simulink model "UnmodifiedMotoHawkModel"  (R2016a)
settings: Solver=ode4  SolverMode=SingleTasking  StartTime=0.0  StopTime=10.0  FixedStep=0.001  RelTol=1e-3
values from neighbouring files (symbols this model uses):
  engineblendfactormap = [0 0 0 0 0 0 0 0 0 0 0 0 ... (420 elements, 21x20)]    [blendfactorvariables.mat]
  motorblendfactormap = [1 1 1 1 1 1 1 1 1 1 1 1 ... (420 elements, 21x20)]    [blendfactorvariables.mat]
  v = [0 5 10 15 20 25 30 35 40 45 50 55 ... (21 elements, 1x21)]    [blendfactorvariables.mat]
  x = [0 1 2 3 4 5 6 7 8 9 10 11 ... (20 elements, 1x20)]    [blendfactorvariables.mat]
undefined symbols (not defined in the file or in its folder): ECU565, motohawk_build_version, motohawk_trunc_name, motohawk_vardec_path
libraries: MotoHawk_lib x58
(part 1 of 2)
settings Model: MotoHawkModelGUID=5F89A2C4-B071-4908-A4AC-2A815C8EF35E  MotoHawkModelOpenTime=2017 4 23 0 12 7.93  MotoHawkBuildVersion=014  MotoHawkBuildStats=struct('TotalFLASH',{0},'TotalEEPROM',{0},'TotalRAM',{0},'AppFLASH',{0},'AppEEPROM',{0},'AppRAM',{0},'HeapRAM',{0},'BuildSuccessCount',{14},'BuildErrorCount',{14})  MotoHawkBuildDirectory=C:\Users\Saumya Trivedi\Documents\MTU\2nd Semester\5750 - Distributed Embedded Control System\Lab\Final Project\Final Models After Testing-20170418T230125Z-001\Final Models After Testing\UnmodifiedMotoHawkModel_Build  MotoHawkBuildInfo=struct('refmodel',{0},'model_name',{'UnmodifiedMotoHawkModel'},'motohawk_version',{'2016a_sp1.1722'},'motohawk_component_version',{'0.0.8'},'motohawk_refmdl_version',{'0.0.1'},'matlab_version',{'9.0.0'},'build_version',{'013'},'module_type',{'ECU565-128'},'layout_type',{'DEV'},'enable_build',{1},'processor_family',{'PPC'},'processor_type',{'MPC565'},'toolchain_vendor',{'gcc-powerpc-eabi'},'toolchain_version',{'4.6.0'},'component',{0},'archive_file',{'PCM128.a'},'fptype',{0},'flash_size',{1048576},'ee_size',{8192},'ram_size',{36864},'decram_size',{4096},'eri_table0_rev',{12},'max_eri_table_size',{65535},'fgnd_base_period_ms',{5},'bgnd_base_period_ms',{50},'build_dir',{'H:\Desktop\5750 Final Project\Final Models\Final Models\UnmodifiedMotoHawkModel_Build'},'dll_name',{'UnmodifiedMotoHawkModel_013'},'srz_name',{'UnmodifiedMotoHawkModel_013'},'fgnd_stack_size',{3072},'fgnd_angle_stack_size',{0},'bgnd_stack_size',{2048},'idle_stack_size',{1024},'irq_stack_size',{1536},'irq_stack_margin',{153},'heap_size',{4096},'heap_margin',{409},'app_int_stack_size',{1024},'shutdown_stack_size',{1024},'use_target_os_config',{0},'target_os',{'Classic ControlCore'},'install_dll_dir',{'C:\ECUFiles\TDBDLL'},'install_srz_dir',{'C:\ECUFiles\Programs'},'mingw_dir',{'C:\Program Files (x86)\Woodward\DevelopmentTools\Toolchains\GCC\win32-pe\4_7_0'},'motohawk_dir',{'C:\Program Files (x86)\Woodward\MCS\MotoHawk\2016a_sp1.1722'},'toolchain_dir',{'C:\Program Files (x86)\Woodward\DevelopmentTools\Toolchains\GCC\powerpc-eabi\4_6_0'},'matlab_root',{'C:\Program Files\MATLAB\R2016a'},'model_guid',{'5F89A2C4-B071-4908-A4AC-2A815C8EF35E'},'build_guid',{'792EB62F-FFF4-451D-B1A3-A5F3AFC705B8'},'token_guid',{'276056F1851C404EAF8E31A6D21D1C4E'})  MotoHawkModelSavedName=UnmodifiedMotoHawkModel  MotoHawkModelElapsedTime=579139.132  MotoHawkBuildGUID=792EB62F-FFF4-451D-B1A3-A5F3AFC705B8  Creator=vaibhav  LastModifiedBy=Saumya Trivedi
settings ConfigSet: Description="This Simulink Configuration Set is preconfigured  for the MotoHawk target \"ECU565-128\"."
settings OptimizationCC: DefaultParameterBehavior=Inlined  InlineInvariantSignals=on  EnhancedBackFolding=on  InitFltsAndDblsToZero=on  NoFixptDivByZeroProtection=on  EfficientFloat2IntCast=on  OptimizeModelRefInitCode=on  LifeSpan=1
settings DebuggingCC: InheritedTsInSrcMsg=none  TasksWithSamePriorityMsg=none  ParameterTunabilityLossMsg=error  ModelReferenceIOMismatchMessage=warning  SFUnexpectedBacktrackingDiag=error  SFNoUnconditionalDefaultTransitionDiag=error
settings HardwareCC: ProdBitPerPointer=32  ProdLargestAtomicInteger=Integer  ProdIntDivRoundTo=Undefined  ProdEndianess=BigEndian  ProdWordSize=32  ProdHWDeviceType=Specified
settings ModelReferenceCC: UpdateModelReferenceTargets=IfOutOfDate  CheckModelReferenceTargetMessage=warning  ModelReferenceNumInstancesAllowed=Single
settings RTWCC: SystemTargetFile=motohawk_ert_rtw.tlc  MakeCommand=make_rtw_motohawk  TemplateMakefile=motohawk_ert_rtw.tmf  Description=MotoHawk(tm) Rapid Prototyping  GenerateReport=on  IncludeHyperlinkInReport=on  LaunchReport=on  GenerateTraceInfo=on  GenerateTraceReport=on  GenerateTraceReportSl=on  GenerateTraceReportSf=on  GenerateTraceReportEml=on
settings CodeAppCC: ForceParamTrailComments=on  IgnoreCustomStorageClasses=off  MaxIdLength=100  OperatorAnnotations=on  SimulinkDataObjDesc=on  SFDataObjDesc=on  MATLABFcnDesc=on  CustomSymbolStrType=$N$R$M  CustomSymbolStrField=$H$N$M  InsertBlockDesc=on  MATLABSourceComments=on  InternalIdentifier=Classic
settings STFCustomTargetCC: TargetLangStandard=C99 (ISO)  ERTMultiwordTypeDef=User defined  ERTMultiwordLength=0  IncludeMdlTerminateFcn=off  GeneratePreprocessorConditionals=Disable all  CombineOutputUpdateFcns=on  SuppressErrorStatus=on  ERTCustomFileBanners=on  SupportContinuousTime=off  SupportNonInlinedSFcns=off  MATLABClassNameForMDSCustomization=Simulink.SoftwareTarget.ERTCustomization  GRTInterface=off  SystemTargetFile=motohawk_ert_rtw.tlc
settings ERTTargetCC: TargetLangStandard=C99 (ISO)  ERTMultiwordTypeDef=User defined  ERTMultiwordLength=0  ParMdlRefBuildCompliant=off  CompOptLevelCompliant=off  ConcurrentExecutionCompliant=off  IncludeMdlTerminateFcn=off  GeneratePreprocessorConditionals=Disable all  SuppressErrorStatus=on  ERTFirstTimeCompliant=off  ModelStepFunctionPrototypeControlCompliant=off  CPPClassGenCompliant=off  UseToolchainInfoCompliant=off  InlinedParameterPlacement=NonHierarchical  ERTCustomFileTemplate=motohawk_file_process.tlc
settings ConfigComp: CovMetricSettings=dwe  CovHtmlReporting=off  CovSaveCumulativeToWorkspaceVar=off  CovSaveSingleToWorkspaceVar=off  CovExternalEMLEnable=on

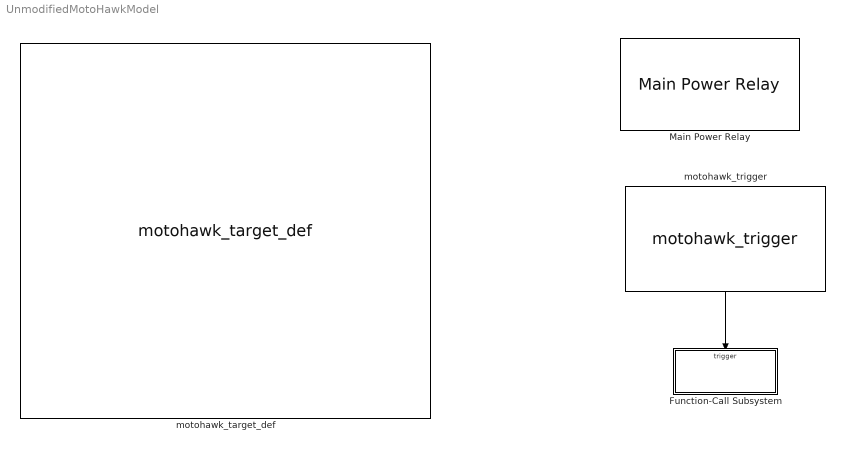
== system UnmodifiedMotoHawkModel ==
  Function-Call Subsystem : Subsystem  TreatAsAtomicUnit=on
  Main Power Relay : MotoHawk_lib/Extra Development Blocks/Main Power Relay  on_delay_count=2  off_delay_count=5  ecup_threshold=100  group='System | Main Power Relay'
  motohawk_target_def : MotoHawk_lib/motohawk_target_def  Priority=-65535  target=ECU565-128  layout=DEV  fptype=single (32 bits)  use_target_os_config=off  target_os=ControlCore  default_target_os=Classic ControlCore  fgnd_stack_size=3*1024  fgnd_angle_stack_size=0  bgnd_stack_size=2*1024  idle_stack_size=1024  irq_stack_size=1536  app_int_stack_size=1024  shutdown_stack_size=1024  heap_size=4*1024  show_margins=off  fgnd_stack_margin=(3*1024) * 0.1  fgnd_angle_stack_margin=0  bgnd_stack_margin=(2*1024) * 0.1  idle_stack_margin=(1024) * 0.1  irq_stack_margin=(1536) * 0.1  app_int_stack_margin=(1024) * 0.1  shutdown_stack_margin=(1024) * 0.1  heap_margin=(4*1024) * 0.1  comp_name=bdroot  comp_img='KVASER_CAN_USB.jpg'  comp_security=No Encryption  comp_build_pass='mhbuild'  comp_sim_pass='mhsim'  comp_multi=off  show_filenames=off  dll_name=motohawk_trunc_name(bdroot, ['_' motohawk_build_version], 50)  srz_name=motohawk_trunc_name(bdroot, ['_' motohawk_build_version], 50)  build_dir='.'  comp_dir='.'
  motohawk_trigger : MotoHawk_lib/Trigger Blocks/motohawk_trigger  Tag=Trigger  Priority=0  trig_name=[]  trigger=FGND_RTI_PERIODIC  priority_order=0  inherited=off  run_disabled=off  override_app_monitor=off  target=ECU565_128
  wires:
  motohawk_trigger/1 -> Function-Call Subsystem/Trigger

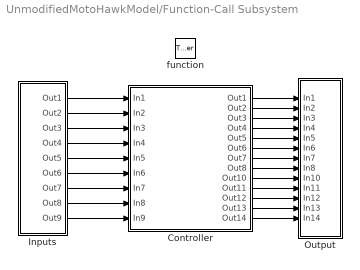
== system UnmodifiedMotoHawkModel/Function-Call Subsystem ==
  function : TriggerPort  TriggerType=function-call  VariantControl=Variant
  Controller : Subsystem
  Inputs : Subsystem
  Output : Subsystem
  wires:
  Inputs/1(Out1) -> Controller/1(In1)
  Inputs/2(Out2) -> Controller/2(In2)
  Inputs/3(Out3) -> Controller/3(In3)
  Inputs/4(Out4) -> Controller/4(In4)
  Inputs/5(Out5) -> Controller/5(In5)
  Inputs/6(Out6) -> Controller/6(In6)
  Inputs/7(Out7) -> Controller/7(In7)
  Inputs/8(Out8) -> Controller/8(In8)
  Inputs/9(Out9) -> Controller/9(In9)
  Controller/1(Out1) -> Output/1(In1)
  Controller/2(Out2) -> Output/2(In2)
  Controller/3(Out3) -> Output/3(In3)
  Controller/4(Out4) -> Output/4(In4)
  Controller/5(Out5) -> Output/5(In5)
  Controller/6(Out6) -> Output/6(In6)
  Controller/7(Out7) -> Output/7(In7)
  Controller/8(Out8) -> Output/8(In8)
  Controller/9(Out10) -> Output/9(In10)
  Controller/10(Out11) -> Output/10(In11)
  Controller/11(Out12) -> Output/11(In12)
  Controller/12(Out13) -> Output/12(In13)
  Controller/13(Out14) -> Output/13(In14)

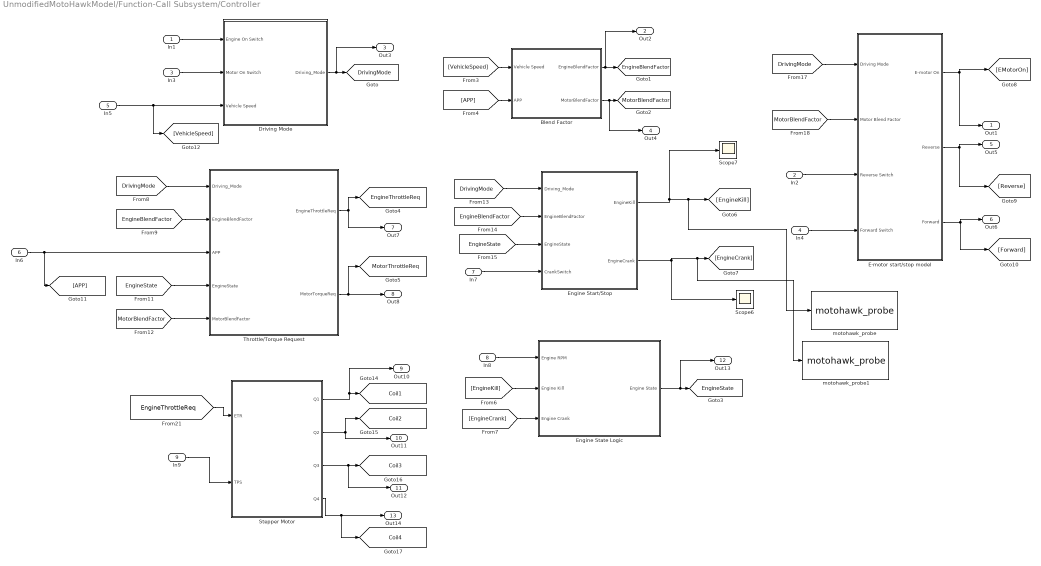
== system UnmodifiedMotoHawkModel/Function-Call Subsystem/Controller ==
  In1 : Inport
  In2 : Inport  Port=2
  In3 : Inport  Port=3
  In4 : Inport  Port=4
  In5 : Inport  Port=5
  In6 : Inport  Port=6
  In7 : Inport  Port=7
  In8 : Inport  Port=8
  In9 : Inport  Port=9
  Blend Factor : Subsystem
  Driving Mode : Subsystem
  E-motor start/stop model : Subsystem
  Engine Start/Stop : Subsystem
  Engine State Logic : Subsystem
  Scope6 : Scope
  Scope7 : Scope
  Stepper Motor : Subsystem
  Throttle/Torque Request : Subsystem
  motohawk_probe : MotoHawk_lib/Calibration & Probing Blocks/motohawk_probe  nam='EngineKill'  show_more=off  name_source=Use Parameter  read_level=1  view_as=Number  enum_struct={'Disabled', 'Enabled'}  vector_style=Wide Row  use_help_units=off  help=''  units=''  use_header_enum=off  row_header_enum={}  col_header_enum={}  use_min_max=off  min_val=-inf  max_val=inf  use_precision=off  precision=''  gain=1  offset=0  exp=1  use_mototune_group=off  mototune_group=motohawk_vardec_path(gcb)
  motohawk_probe1 : MotoHawk_lib/Calibration & Probing Blocks/motohawk_probe  nam='EngineCrank'  show_more=off  name_source=Use Parameter  read_level=1  view_as=Number  enum_struct={'Disabled', 'Enabled'}  vector_style=Wide Row  use_help_units=off  help=''  units=''  use_header_enum=off  row_header_enum={}  col_header_enum={}  use_min_max=off  min_val=-inf  max_val=inf  use_precision=off  precision=''  gain=1  offset=0  exp=1  use_mototune_group=off  mototune_group=motohawk_vardec_path(gcb)
  Out1 : Outport
  Out2 : Outport  Port=2
  Out3 : Outport  Port=3
  Out4 : Outport  Port=4
  Out5 : Outport  Port=5
  Out6 : Outport  Port=6
  Out7 : Outport  Port=7
  Out8 : Outport  Port=8
  Out10 : Outport  Port=9
  Out11 : Outport  Port=10
  Out12 : Outport  Port=11
  Out13 : Outport  Port=12
  Out14 : Outport  Port=13
  tag scope: Coil1=global, Coil2=global, Coil3=global, Coil4=global, DrivingMode=global, EngineBlendFactor=global, EngineState=global, EngineThrottleReq=global, MotorBlendFactor=global, MotorThrottleReq=global
  wires:
  Driving Mode/1(Driving_Mode) -> Out3/1, [DrivingMode]
  [VehicleSpeed] -> Blend Factor/1(Vehicle Speed)
  [APP] -> Blend Factor/2(APP)
  Blend Factor/2(MotorBlendFactor) -> Out4/1, [MotorBlendFactor]
  [EngineCrank] -> Engine State Logic/3(Engine Crank)
  [EngineKill] -> Engine State Logic/2(Engine Kill)
  Engine State Logic/1(Engine State) -> Out13/1, [EngineState]
  [DrivingMode] -> Throttle/Torque Request/1(Driving_Mode)
  [EngineBlendFactor] -> Throttle/Torque Request/2(EngineBlendFactor)
  Blend Factor/1(EngineBlendFactor) -> Out2/1, [EngineBlendFactor]
  E-motor start/stop model/2(Reverse) -> Out5/1, [Reverse]
  E-motor start/stop model/1(E-motor On) -> [EMotorOn], Out1/1
  [EngineState] -> Throttle/Torque Request/4(EngineState)
  [MotorBlendFactor] -> Throttle/Torque Request/5(MotorBlendFactor)
  Throttle/Torque Request/1(EngineThrottleReq) -> Out7/1, [EngineThrottleReq]
  Throttle/Torque Request/2(MotorTorqueReq) -> [MotorThrottleReq], Out8/1
  [DrivingMode] -> Engine Start/Stop/1(Driving_Mode)
  [EngineBlendFactor] -> Engine Start/Stop/2(EngineBlendFactor)
  [EngineState] -> Engine Start/Stop/3(EngineState)
  Engine Start/Stop/1(EngineKill) -> Scope7/1, motohawk_probe/1, [EngineKill]
  [DrivingMode] -> E-motor start/stop model/1(Driving Mode)
  E-motor start/stop model/3(Forward) -> Out6/1, [Forward]
  [EngineThrottleReq] -> Stepper Motor/1(ETR)
  Stepper Motor/1(Q1) -> Out10/1, [Coil1]
  Stepper Motor/4(Q4) -> [Coil4], Out14/1
  Stepper Motor/3(Q3) -> Out12/1, [Coil3]
  Stepper Motor/2(Q2) -> [Coil2], Out11/1
  [MotorBlendFactor] -> E-motor start/stop model/2(Motor Blend Factor)
  Engine Start/Stop/2(EngineCrank) -> motohawk_probe1/1, [EngineCrank], Scope6/1
  In4/1 -> E-motor start/stop model/4(Forward Switch)
  In2/1 -> E-motor start/stop model/3(Reverse Switch)
  In3/1 -> Driving Mode/2(Motor On Switch)
  In1/1 -> Driving Mode/1(Engine On Switch)
  In9/1 -> Stepper Motor/2(TPS)
  In8/1 -> Engine State Logic/1(Engine RPM)
  In7/1 -> Engine Start/Stop/4(CrankSwitch)
  In5/1 -> [VehicleSpeed], Driving Mode/3(Vehicle Speed)
  In6/1 -> Throttle/Torque Request/3(APP), [APP]

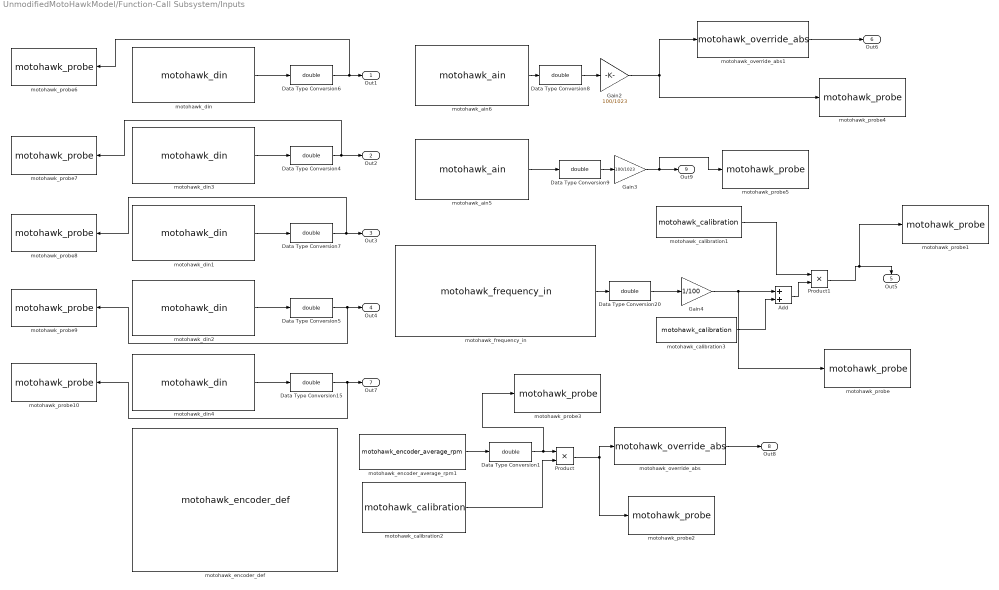
== system UnmodifiedMotoHawkModel/Function-Call Subsystem/Inputs ==
  Add : Sum
  Data Type Conversion{1,4..9,15,20} (9 alike) : DataTypeConversion  OutDataTypeStr=double
  Gain2 : Gain  Gain=100/1023
  Gain3 : Gain  Gain=100/1023
  Gain4 : Gain  Gain=1/100
  Product : Product
  Product1 : Product
  motohawk_ain5 : MotoHawk_lib/Analog I//O Blocks/motohawk_ain  res_name=['TPS']  text_resource=AN25M  code_resource=NONE  val_resource=-1  target=ECU565-128  resource_enum_str=(None)=-1,ECUP=53,DRVP=54,XDRP=55,AN1M=56,AN2M=57,AN3M=58,AN4M=59,AN5M=60,AN6M=61,AN7M=62,AN8M=63,AN9M=64,AN10M=65,AN11M=66,AN12M=67,AN13M=68,AN14M=69,AN15M=70,AN16M=71,AN17M=72,AN18M=73,AN19M=74,AN20M=75,AN21M=76,AN22M=77,AN23M=78,AN24M=79,AN25M=80,AN26M=81,AN27M=82,AN28M=83,AN29M=84,AN30M=85,AN31M=86,AN32M=87,AN33M=88,AN34M=89,O2A=90,O2B=91,XDRP_B=92,REF_14V=143  altref=5V Reference  typ=uint16  num_adc_bits=10  use_stat=off  use_vardec=off  nam='RTD1_MW'  read_level=1  write_level=1  group='System | I/O Pins | Inputs Config'
  motohawk_ain6 : MotoHawk_lib/Analog I//O Blocks/motohawk_ain  res_name=['APP']  text_resource=AN22M  code_resource=NONE  val_resource=-1  target=ECU565-128  resource_enum_str=(None)=-1,ECUP=53,DRVP=54,XDRP=55,AN1M=56,AN2M=57,AN3M=58,AN4M=59,AN5M=60,AN6M=61,AN7M=62,AN8M=63,AN9M=64,AN10M=65,AN11M=66,AN12M=67,AN13M=68,AN14M=69,AN15M=70,AN16M=71,AN17M=72,AN18M=73,AN19M=74,AN20M=75,AN21M=76,AN22M=77,AN23M=78,AN24M=79,AN25M=80,AN26M=81,AN27M=82,AN28M=83,AN29M=84,AN30M=85,AN31M=86,AN32M=87,AN33M=88,AN34M=89,O2A=90,O2B=91,XDRP_B=92,REF_14V=143  altref=5V Reference  typ=uint16  num_adc_bits=10  use_stat=off  use_vardec=off  nam='RTD1_MW'  read_level=1  write_level=1  group='System | I/O Pins | Inputs Config'
  motohawk_calibration1 : MotoHawk_lib/Calibration & Probing Blocks/motohawk_calibration  nam='Speed_Gain'  val=1  storage=Calibration  show_more=off  name_source=Use Parameter  data_type=Inherit from 'Default Value'  read_level=1  write_level=1  ovr_cals=on  view_as=Number  enum_struct={'Disabled', 'Enabled'}  vector_style=Wide Row  use_help_units=off  help=''  units=''  use_header_enum=off  row_header_enum={}  col_header_enum={}  use_min_max=off  min_val=-inf  max_val=inf  use_precision=off  precision=''  gain=1  offset=0  exp=1  use_mototune_group=off  mototune_group=motohawk_vardec_path(gcb)  data_stores=motohawk_sfun_calibration_data_stores
  motohawk_calibration2 : MotoHawk_lib/Calibration & Probing Blocks/motohawk_calibration  nam='Rpm_Gain'  val=1  storage=Calibration  show_more=off  name_source=Use Parameter  data_type=Inherit from 'Default Value'  read_level=1  write_level=1  ovr_cals=on  view_as=Number  enum_struct={'Disabled', 'Enabled'}  vector_style=Wide Row  use_help_units=off  help=''  units=''  use_header_enum=off  row_header_enum={}  col_header_enum={}  use_min_max=off  min_val=-inf  max_val=inf  use_precision=off  precision=''  gain=1  offset=0  exp=1  use_mototune_group=off  mototune_group=motohawk_vardec_path(gcb)  data_stores=motohawk_sfun_calibration_data_stores
  motohawk_calibration3 : MotoHawk_lib/Calibration & Probing Blocks/motohawk_calibration  nam='Speed_Offset'  val=1  storage=Calibration  show_more=off  name_source=Use Parameter  data_type=Inherit from 'Default Value'  read_level=1  write_level=1  ovr_cals=on  view_as=Number  enum_struct={'Disabled', 'Enabled'}  vector_style=Wide Row  use_help_units=off  help=''  units=''  use_header_enum=off  row_header_enum={}  col_header_enum={}  use_min_max=off  min_val=-inf  max_val=inf  use_precision=off  precision=''  gain=1  offset=0  exp=1  use_mototune_group=off  mototune_group=motohawk_vardec_path(gcb)  data_stores=motohawk_sfun_calibration_data_stores
  motohawk_din : MotoHawk_lib/Digital I//O Blocks/motohawk_din  resource_name=['EngineOnSwitch']  text_resource=AN5M  code_resource=NONE  val_resource=-1  target=ECU565-128  resource_enum_str=(None)=-1,AN1M=56,AN2M=57,AN3M=58,AN4M=59,AN5M=60,AN6M=61,AN7M=62,AN8M=63,AN9M=64,AN10M=65,AN11M=66,AN12M=67,AN13M=68,AN14M=69,AN15M=70,AN16M=71,AN17M=72,AN18M=73,AN19M=74,AN20M=75,AN21M=76,AN22M=77,AN23M=78,AN24M=79,AN25M=80,AN26M=81,AN27M=82,AN28M=83,AN29M=84,AN30M=85,AN31M=86,AN32M=87,AN33M=88,AN34M=89,O2A=90,O2B=91,DG1M=93,DG2M=94,DG3M=95,DG4M=96,DG5M=102,DG6M=103,DG7M=104,SPD1=105,SPD2=106,DG8M=111  pullup=None  use_stat=off  use_vardec=off  nam=[]  read_level=1  write_level=1  group='System | I/O Pins | Inputs Config'
  motohawk_din1 : MotoHawk_lib/Digital I//O Blocks/motohawk_din  resource_name=['MotorOnSwitch']  text_resource=AN6M  code_resource=NONE  val_resource=-1  target=ECU565-128  resource_enum_str=(None)=-1,AN1M=56,AN2M=57,AN3M=58,AN4M=59,AN5M=60,AN6M=61,AN7M=62,AN8M=63,AN9M=64,AN10M=65,AN11M=66,AN12M=67,AN13M=68,AN14M=69,AN15M=70,AN16M=71,AN17M=72,AN18M=73,AN19M=74,AN20M=75,AN21M=76,AN22M=77,AN23M=78,AN24M=79,AN25M=80,AN26M=81,AN27M=82,AN28M=83,AN29M=84,AN30M=85,AN31M=86,AN32M=87,AN33M=88,AN34M=89,O2A=90,O2B=91,DG1M=93,DG2M=94,DG3M=95,DG4M=96,DG5M=102,DG6M=103,DG7M=104,SPD1=105,SPD2=106,DG8M=111  pullup=None  use_stat=off  use_vardec=off  nam=[]  read_level=1  write_level=1  group='System | I/O Pins | Inputs Config'
  motohawk_din2 : MotoHawk_lib/Digital I//O Blocks/motohawk_din  resource_name=['Forward_Switch']  text_resource=AN1M  code_resource=NONE  val_resource=-1  target=ECU565-128  resource_enum_str=(None)=-1,AN1M=56,AN2M=57,AN3M=58,AN4M=59,AN5M=60,AN6M=61,AN7M=62,AN8M=63,AN9M=64,AN10M=65,AN11M=66,AN12M=67,AN13M=68,AN14M=69,AN15M=70,AN16M=71,AN17M=72,AN18M=73,AN19M=74,AN20M=75,AN21M=76,AN22M=77,AN23M=78,AN24M=79,AN25M=80,AN26M=81,AN27M=82,AN28M=83,AN29M=84,AN30M=85,AN31M=86,AN32M=87,AN33M=88,AN34M=89,O2A=90,O2B=91,DG1M=93,DG2M=94,DG3M=95,DG4M=96,DG5M=102,DG6M=103,DG7M=104,SPD1=105,SPD2=106,DG8M=111  pullup=None  use_stat=off  use_vardec=off  nam=[]  read_level=1  write_level=1  group='System | I/O Pins | Inputs Config'
  motohawk_din3 : MotoHawk_lib/Digital I//O Blocks/motohawk_din  resource_name=['Reverse_Switch']  text_resource=AN3M  code_resource=NONE  val_resource=-1  target=ECU565-128  resource_enum_str=(None)=-1,AN1M=56,AN2M=57,AN3M=58,AN4M=59,AN5M=60,AN6M=61,AN7M=62,AN8M=63,AN9M=64,AN10M=65,AN11M=66,AN12M=67,AN13M=68,AN14M=69,AN15M=70,AN16M=71,AN17M=72,AN18M=73,AN19M=74,AN20M=75,AN21M=76,AN22M=77,AN23M=78,AN24M=79,AN25M=80,AN26M=81,AN27M=82,AN28M=83,AN29M=84,AN30M=85,AN31M=86,AN32M=87,AN33M=88,AN34M=89,O2A=90,O2B=91,DG1M=93,DG2M=94,DG3M=95,DG4M=96,DG5M=102,DG6M=103,DG7M=104,SPD1=105,SPD2=106,DG8M=111  pullup=None  use_stat=off  use_vardec=off  nam=[]  read_level=1  write_level=1  group='System | I/O Pins | Inputs Config'
  motohawk_din4 : MotoHawk_lib/Digital I//O Blocks/motohawk_din  resource_name=['CrankSwitch']  text_resource=AN9M  code_resource=NONE  val_resource=-1  target=ECU565-128  resource_enum_str=(None)=-1,AN1M=56,AN2M=57,AN3M=58,AN4M=59,AN5M=60,AN6M=61,AN7M=62,AN8M=63,AN9M=64,AN10M=65,AN11M=66,AN12M=67,AN13M=68,AN14M=69,AN15M=70,AN16M=71,AN17M=72,AN18M=73,AN19M=74,AN20M=75,AN21M=76,AN22M=77,AN23M=78,AN24M=79,AN25M=80,AN26M=81,AN27M=82,AN28M=83,AN29M=84,AN30M=85,AN31M=86,AN32M=87,AN33M=88,AN34M=89,O2A=90,O2B=91,DG1M=93,DG2M=94,DG3M=95,DG4M=96,DG5M=102,DG6M=103,DG7M=104,SPD1=105,SPD2=106,DG8M=111  pullup=None  use_stat=off  use_vardec=off  nam=[]  read_level=1  write_level=1  group='System | I/O Pins | Inputs Config'
  motohawk_encoder_average_rpm1 : MotoHawk_lib/Encoder Blocks/motohawk_encoder_average_rpm  resolution=1
  motohawk_encoder_def : MotoHawk_lib/Encoder Blocks/motohawk_encoder_def  encoder_type=36 Minus 1 - 4-Stroke - No CAM  interface=Digital Crank  sync=Falling Edge  crnkpullup=Weak Pullup  camsync=Rising Edge  campullup=Weak Pullup  angle_offset=0  sec_tdcoffset=0  cam_delay=0  teeth_after_cam=-1  ignore_teeth=0  ignore_delay=0  angles=[0 360 180 540]  cnk_align_with_cam=off  adaptive_vr_cnk=off  adaptive_vr_cam=on  cal_cylinders=on  max_cylinders=8  num_cylinders=4  read_level=1  write_level=1  ovr_cals=on  group='System | Encoder'
  motohawk_frequency_in : MotoHawk_lib/Advanced Digital I//O/motohawk_frequency_in  res_name=['VehicleSpeed']  text_resource=SPD1  code_resource=NONE  val_resource=-1  target=ECU565-128  resource_enum_str=(None)=-1,DG1M=93,DG2M=94,DG3M=95,DG4M=96,DG5M=102,DG6M=103,DG7M=104,SPD1=105,SPD2=106,DG8M=111  edge=Rising Edge  alias=Disabled  min_freq=100  sig=Digital Input  ipwm=No Duty Cycle Measurement  itrig=off  Nmax=10  use_avg=off  avg_mode=Fixed Interval  fixed_avg_pulses=2  use_vardec=off  use_cal=off  nam=[]  read_level=1  write_level=1  group='System | I/O Pins | Inputs Config'  cal_group='System | I/O Pins | Frequency In Config'
  motohawk_override_abs : MotoHawk_lib/Calibration & Probing Blocks/motohawk_override_abs  parent_name='Engine_Override'  parent_val=0  show_more=off  name_source=Use Parameter  parent_read_level=1  parent_override_level=1  view_as=Number  enum_struct={'Disabled', 'Enabled'}  use_help_units=off  parent_help=''  parent_units=''  use_min_max=off  parent_min=-inf  parent_max=inf  use_precision=off  parent_precision=''  parent_gain=1  parent_offset=0  parent_exp=1  use_mototune_group=off  parent_group=motohawk_vardec_path(gcb)
  motohawk_override_abs1 : MotoHawk_lib/Calibration & Probing Blocks/motohawk_override_abs  parent_name='APP_Override'  parent_val=0  show_more=off  name_source=Use Parameter  parent_read_level=1  parent_override_level=1  view_as=Number  enum_struct={'Disabled', 'Enabled'}  use_help_units=off  parent_help=''  parent_units=''  use_min_max=off  parent_min=-inf  parent_max=inf  use_precision=off  parent_precision=''  parent_gain=1  parent_offset=0  parent_exp=1  use_mototune_group=off  parent_group=motohawk_vardec_path(gcb)
  motohawk_probe : MotoHawk_lib/Calibration & Probing Blocks/motohawk_probe  nam='Frequency'  show_more=off  name_source=Use Parameter  read_level=1  view_as=Number  enum_struct={'Disabled', 'Enabled'}  vector_style=Wide Row  use_help_units=off  help=''  units=''  use_header_enum=off  row_header_enum={}  col_header_enum={}  use_min_max=off  min_val=-inf  max_val=inf  use_precision=off  precision=''  gain=1  offset=0  exp=1  use_mototune_group=off  mototune_group=motohawk_vardec_path(gcb)
  motohawk_probe1 : MotoHawk_lib/Calibration & Probing Blocks/motohawk_probe  nam='Speed'  show_more=off  name_source=Use Parameter  read_level=1  view_as=Number  enum_struct={'Disabled', 'Enabled'}  vector_style=Wide Row  use_help_units=off  help=''  units=''  use_header_enum=off  row_header_enum={}  col_header_enum={}  use_min_max=off  min_val=-inf  max_val=inf  use_precision=off  precision=''  gain=1  offset=0  exp=1  use_mototune_group=off  mototune_group=motohawk_vardec_path(gcb)
  motohawk_probe10 : MotoHawk_lib/Calibration & Probing Blocks/motohawk_probe  nam='CrankSwitch'  show_more=off  name_source=Use Parameter  read_level=1  view_as=Number  enum_struct={'Disabled', 'Enabled'}  vector_style=Wide Row  use_help_units=off  help=''  units=''  use_header_enum=off  row_header_enum={}  col_header_enum={}  use_min_max=off  min_val=-inf  max_val=inf  use_precision=off  precision=''  gain=1  offset=0  exp=1  use_mototune_group=off  mototune_group=motohawk_vardec_path(gcb)
  motohawk_probe2 : MotoHawk_lib/Calibration & Probing Blocks/motohawk_probe  nam='Engine_RPM'  show_more=off  name_source=Use Parameter  read_level=1  view_as=Number  enum_struct={'Disabled', 'Enabled'}  vector_style=Wide Row  use_help_units=off  help=''  units=''  use_header_enum=off  row_header_enum={}  col_header_enum={}  use_min_max=off  min_val=-inf  max_val=inf  use_precision=off  precision=''  gain=1  offset=0  exp=1  use_mototune_group=off  mototune_group=motohawk_vardec_path(gcb)
  motohawk_probe3 : MotoHawk_lib/Calibration & Probing Blocks/motohawk_probe  nam='Input_Engine_RPM'  show_more=off  name_source=Use Parameter  read_level=1  view_as=Number  enum_struct={'Disabled', 'Enabled'}  vector_style=Wide Row  use_help_units=off  help=''  units=''  use_header_enum=off  row_header_enum={}  col_header_enum={}  use_min_max=off  min_val=-inf  max_val=inf  use_precision=off  precision=''  gain=1  offset=0  exp=1  use_mototune_group=off  mototune_group=motohawk_vardec_path(gcb)
  motohawk_probe4 : MotoHawk_lib/Calibration & Probing Blocks/motohawk_probe  nam='APP'  show_more=off  name_source=Use Parameter  read_level=1  view_as=Number  enum_struct={'Disabled', 'Enabled'}  vector_style=Wide Row  use_help_units=off  help=''  units=''  use_header_enum=off  row_header_enum={}  col_header_enum={}  use_min_max=off  min_val=-inf  max_val=inf  use_precision=off  precision=''  gain=1  offset=0  exp=1  use_mototune_group=off  mototune_group=motohawk_vardec_path(gcb)
  motohawk_probe5 : MotoHawk_lib/Calibration & Probing Blocks/motohawk_probe  nam='TPS'  show_more=off  name_source=Use Parameter  read_level=1  view_as=Number  enum_struct={'Disabled', 'Enabled'}  vector_style=Wide Row  use_help_units=off  help=''  units=''  use_header_enum=off  row_header_enum={}  col_header_enum={}  use_min_max=off  min_val=-inf  max_val=inf  use_precision=off  precision=''  gain=1  offset=0  exp=1  use_mototune_group=off  mototune_group=motohawk_vardec_path(gcb)
  motohawk_probe6 : MotoHawk_lib/Calibration & Probing Blocks/motohawk_probe  nam='EngineOnSwitch'  show_more=off  name_source=Use Parameter  read_level=1  view_as=Number  enum_struct={'Disabled', 'Enabled'}  vector_style=Wide Row  use_help_units=off  help=''  units=''  use_header_enum=off  row_header_enum={}  col_header_enum={}  use_min_max=off  min_val=-inf  max_val=inf  use_precision=off  precision=''  gain=1  offset=0  exp=1  use_mototune_group=off  mototune_group=motohawk_vardec_path(gcb)
  motohawk_probe7 : MotoHawk_lib/Calibration & Probing Blocks/motohawk_probe  nam='Reverse_Switch'  show_more=off  name_source=Use Parameter  read_level=1  view_as=Number  enum_struct={'Disabled', 'Enabled'}  vector_style=Wide Row  use_help_units=off  help=''  units=''  use_header_enum=off  row_header_enum={}  col_header_enum={}  use_min_max=off  min_val=-inf  max_val=inf  use_precision=off  precision=''  gain=1  offset=0  exp=1  use_mototune_group=off  mototune_group=motohawk_vardec_path(gcb)
  motohawk_probe8 : MotoHawk_lib/Calibration & Probing Blocks/motohawk_probe  nam='MotorOnSwitch'  show_more=off  name_source=Use Parameter  read_level=1  view_as=Number  enum_struct={'Disabled', 'Enabled'}  vector_style=Wide Row  use_help_units=off  help=''  units=''  use_header_enum=off  row_header_enum={}  col_header_enum={}  use_min_max=off  min_val=-inf  max_val=inf  use_precision=off  precision=''  gain=1  offset=0  exp=1  use_mototune_group=off  mototune_group=motohawk_vardec_path(gcb)
  motohawk_probe9 : MotoHawk_lib/Calibration & Probing Blocks/motohawk_probe  nam='ForwardSwitch'  show_more=off  name_source=Use Parameter  read_level=1  view_as=Number  enum_struct={'Disabled', 'Enabled'}  vector_style=Wide Row  use_help_units=off  help=''  units=''  use_header_enum=off  row_header_enum={}  col_header_enum={}  use_min_max=off  min_val=-inf  max_val=inf  use_precision=off  precision=''  gain=1  offset=0  exp=1  use_mototune_group=off  mototune_group=motohawk_vardec_path(gcb)
  Out1 : Outport
  Out2 : Outport  Port=2
  Out3 : Outport  Port=3
  Out4 : Outport  Port=4
  Out5 : Outport  Port=5
  Out6 : Outport  Port=6
  Out7 : Outport  Port=7
  Out8 : Outport  Port=8
  Out9 : Outport  Port=9
  wires:
  motohawk_din/1 -> Data Type Conversion6/1
  motohawk_din1/1 -> Data Type Conversion7/1
  motohawk_override_abs/1 -> Out8/1
  Data Type Conversion6/1 -> motohawk_probe6/1, Out1/1
  motohawk_ain6/1 -> Data Type Conversion8/1
  motohawk_encoder_average_rpm1/1 -> Data Type Conversion1/1
  Data Type Conversion1/1 -> motohawk_probe3/1, Product/1
  Product/1 -> motohawk_override_abs/1, motohawk_probe2/1
  motohawk_calibration2/1 -> Product/2
  Gain2/1 -> motohawk_probe4/1, motohawk_override_abs1/1
  motohawk_ain5/1 -> Data Type Conversion9/1
  Gain3/1 -> motohawk_probe5/1, Out9/1
  Data Type Conversion15/1 -> motohawk_probe10/1, Out7/1
  Data Type Conversion4/1 -> motohawk_probe7/1, Out2/1
  Data Type Conversion5/1 -> motohawk_probe9/1, Out4/1
  Data Type Conversion8/1 -> Gain2/1
  Data Type Conversion9/1 -> Gain3/1
  Product1/1 -> motohawk_probe1/1, Out5/1
  Data Type Conversion20/1 -> Gain4/1
  motohawk_din4/1 -> Data Type Conversion15/1
  motohawk_din3/1 -> Data Type Conversion4/1
  motohawk_din2/1 -> Data Type Conversion5/1
  Data Type Conversion7/1 -> motohawk_probe8/1, Out3/1
  motohawk_calibration3/1 -> Add/2
  Add/1 -> Product1/2
  motohawk_calibration1/1 -> Product1/1
  motohawk_frequency_in/1 -> Data Type Conversion20/1
  Gain4/1 -> motohawk_probe/1, Add/1
  motohawk_override_abs1/1 -> Out6/1

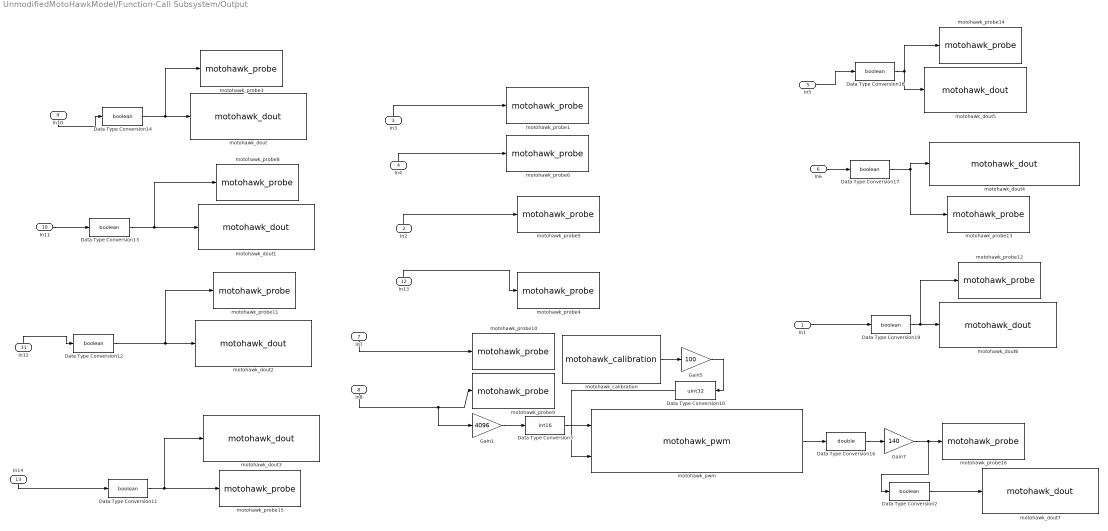
== system UnmodifiedMotoHawkModel/Function-Call Subsystem/Output ==
  In1 : Inport
  In2 : Inport  Port=2
  In3 : Inport  Port=3
  In4 : Inport  Port=4
  In5 : Inport  Port=5
  In6 : Inport  Port=6
  In7 : Inport  Port=7
  In8 : Inport  Port=8
  In10 : Inport  Port=9
  In11 : Inport  Port=10
  In12 : Inport  Port=11
  In13 : Inport  Port=12
  In14 : Inport  Port=13
  Data Type Conversion10 : DataTypeConversion  OutDataTypeStr=uint32
  Data Type Conversion{2,11..14,17..19} (8 alike) : DataTypeConversion  OutDataTypeStr=boolean
  Data Type Conversion16 : DataTypeConversion  OutDataTypeStr=double
  Data Type Conversion3 : DataTypeConversion  OutDataTypeStr=int16
  Gain1 : Gain  Gain=4096
  Gain5 : Gain  Gain=100
  Gain7 : Gain  Gain=140
  motohawk_calibration : MotoHawk_lib/Calibration & Probing Blocks/motohawk_calibration  nam='PWMFrequency'  val=0  storage=Calibration  show_more=off  name_source=Use Parameter  data_type=Inherit from 'Default Value'  read_level=1  write_level=1  ovr_cals=on  view_as=Number  enum_struct={'Disabled', 'Enabled'}  vector_style=Wide Row  use_help_units=off  help=''  units=''  use_header_enum=off  row_header_enum={}  col_header_enum={}  use_min_max=off  min_val=-inf  max_val=inf  use_precision=off  precision=''  gain=1  offset=0  exp=1  use_mototune_group=off  mototune_group=motohawk_vardec_path(gcb)  data_stores=motohawk_sfun_calibration_data_stores
  motohawk_dout : MotoHawk_lib/Digital I//O Blocks/motohawk_dout  resource_name=['Coil1']  text_resource=LSD5  target=ECU565-128  use_diag=off  use_vardec=off  nam=[]  read_level=1  write_level=1  group='System | I/O Pins | Outputs Config'
  motohawk_dout1 : MotoHawk_lib/Digital I//O Blocks/motohawk_dout  resource_name=['Coil2']  text_resource=LSD6  target=ECU565-128  use_diag=off  use_vardec=off  nam=[]  read_level=1  write_level=1  group='System | I/O Pins | Outputs Config'
  motohawk_dout2 : MotoHawk_lib/Digital I//O Blocks/motohawk_dout  resource_name=['Coil3']  text_resource=LSD7  target=ECU565-128  use_diag=off  use_vardec=off  nam=[]  read_level=1  write_level=1  group='System | I/O Pins | Outputs Config'
  motohawk_dout3 : MotoHawk_lib/Digital I//O Blocks/motohawk_dout  resource_name=['Coil4']  text_resource=LSD8  target=ECU565-128  use_diag=off  use_vardec=off  nam=[]  read_level=1  write_level=1  group='System | I/O Pins | Outputs Config'
  motohawk_dout4 : MotoHawk_lib/Digital I//O Blocks/motohawk_dout  resource_name=['Forward']  text_resource=LSD2  target=ECU565-128  use_diag=off  use_vardec=off  nam=[]  read_level=1  write_level=1  group='System | I/O Pins | Outputs Config'
  motohawk_dout5 : MotoHawk_lib/Digital I//O Blocks/motohawk_dout  resource_name=['Reverse']  text_resource=LSD3  target=ECU565-128  use_diag=off  use_vardec=off  nam=[]  read_level=1  write_level=1  group='System | I/O Pins | Outputs Config'
  motohawk_dout6 : MotoHawk_lib/Digital I//O Blocks/motohawk_dout  resource_name=['EmotorOn']  text_resource=LSD4  target=ECU565-128  use_diag=off  use_vardec=off  nam=[]  read_level=1  write_level=1  group='System | I/O Pins | Outputs Config'
  motohawk_dout7 : MotoHawk_lib/Digital I//O Blocks/motohawk_dout  resource_name=['EMotorVoltage']  text_resource=EST 1  target=ECU565-128  use_diag=off  use_vardec=off  nam=[]  read_level=1  write_level=1  group='System | I/O Pins | Outputs Config'
  motohawk_probe1 : MotoHawk_lib/Calibration & Probing Blocks/motohawk_probe  nam='DrivingMode'  show_more=off  name_source=Use Parameter  read_level=1  view_as=Number  enum_struct={'Disabled', 'Enabled'}  vector_style=Wide Row  use_help_units=off  help=''  units=''  use_header_enum=off  row_header_enum={}  col_header_enum={}  use_min_max=off  min_val=-inf  max_val=inf  use_precision=off  precision=''  gain=1  offset=0  exp=1  use_mototune_group=off  mototune_group=motohawk_vardec_path(gcb)
  motohawk_probe10 : MotoHawk_lib/Calibration & Probing Blocks/motohawk_probe  nam='EngineThrottleReq'  show_more=off  name_source=Use Parameter  read_level=1  view_as=Number  enum_struct={'Disabled', 'Enabled'}  vector_style=Wide Row  use_help_units=off  help=''  units=''  use_header_enum=off  row_header_enum={}  col_header_enum={}  use_min_max=off  min_val=-inf  max_val=inf  use_precision=off  precision=''  gain=1  offset=0  exp=1  use_mototune_group=off  mototune_group=motohawk_vardec_path(gcb)
  motohawk_probe11 : MotoHawk_lib/Calibration & Probing Blocks/motohawk_probe  nam='Coil3'  show_more=off  name_source=Use Parameter  read_level=1  view_as=Number  enum_struct={'Disabled', 'Enabled'}  vector_style=Wide Row  use_help_units=off  help=''  units=''  use_header_enum=off  row_header_enum={}  col_header_enum={}  use_min_max=off  min_val=-inf  max_val=inf  use_precision=off  precision=''  gain=1  offset=0  exp=1  use_mototune_group=off  mototune_group=motohawk_vardec_path(gcb)
  motohawk_probe12 : MotoHawk_lib/Calibration & Probing Blocks/motohawk_probe  nam='EmotorOn'  show_more=off  name_source=Use Parameter  read_level=1  view_as=Number  enum_struct={'Disabled', 'Enabled'}  vector_style=Wide Row  use_help_units=off  help=''  units=''  use_header_enum=off  row_header_enum={}  col_header_enum={}  use_min_max=off  min_val=-inf  max_val=inf  use_precision=off  precision=''  gain=1  offset=0  exp=1  use_mototune_group=off  mototune_group=motohawk_vardec_path(gcb)
  motohawk_probe13 : MotoHawk_lib/Calibration & Probing Blocks/motohawk_probe  nam='Forward'  show_more=off  name_source=Use Parameter  read_level=1  view_as=Number  enum_struct={'Disabled', 'Enabled'}  vector_style=Wide Row  use_help_units=off  help=''  units=''  use_header_enum=off  row_header_enum={}  col_header_enum={}  use_min_max=off  min_val=-inf  max_val=inf  use_precision=off  precision=''  gain=1  offset=0  exp=1  use_mototune_group=off  mototune_group=motohawk_vardec_path(gcb)
  motohawk_probe14 : MotoHawk_lib/Calibration & Probing Blocks/motohawk_probe  nam='Reverse'  show_more=off  name_source=Use Parameter  read_level=1  view_as=Number  enum_struct={'Disabled', 'Enabled'}  vector_style=Wide Row  use_help_units=off  help=''  units=''  use_header_enum=off  row_header_enum={}  col_header_enum={}  use_min_max=off  min_val=-inf  max_val=inf  use_precision=off  precision=''  gain=1  offset=0  exp=1  use_mototune_group=off  mototune_group=motohawk_vardec_path(gcb)
  motohawk_probe15 : MotoHawk_lib/Calibration & Probing Blocks/motohawk_probe  nam='Coil4'  show_more=off  name_source=Use Parameter  read_level=1  view_as=Number  enum_struct={'Disabled', 'Enabled'}  vector_style=Wide Row  use_help_units=off  help=''  units=''  use_header_enum=off  row_header_enum={}  col_header_enum={}  use_min_max=off  min_val=-inf  max_val=inf  use_precision=off  precision=''  gain=1  offset=0  exp=1  use_mototune_group=off  mototune_group=motohawk_vardec_path(gcb)
  motohawk_probe16 : MotoHawk_lib/Calibration & Probing Blocks/motohawk_probe  nam='EMotorVoltage'  show_more=off  name_source=Use Parameter  read_level=1  view_as=Number  enum_struct={'Disabled', 'Enabled'}  vector_style=Wide Row  use_help_units=off  help=''  units=''  use_header_enum=off  row_header_enum={}  col_header_enum={}  use_min_max=off  min_val=-inf  max_val=inf  use_precision=off  precision=''  gain=1  offset=0  exp=1  use_mototune_group=off  mototune_group=motohawk_vardec_path(gcb)
  motohawk_probe3 : MotoHawk_lib/Calibration & Probing Blocks/motohawk_probe  nam='Coil1'  show_more=off  name_source=Use Parameter  read_level=1  view_as=Number  enum_struct={'Disabled', 'Enabled'}  vector_style=Wide Row  use_help_units=off  help=''  units=''  use_header_enum=off  row_header_enum={}  col_header_enum={}  use_min_max=off  min_val=-inf  max_val=inf  use_precision=off  precision=''  gain=1  offset=0  exp=1  use_mototune_group=off  mototune_group=motohawk_vardec_path(gcb)
  motohawk_probe4 : MotoHawk_lib/Calibration & Probing Blocks/motohawk_probe  nam='EngineState'  show_more=off  name_source=Use Parameter  read_level=1  view_as=Number  enum_struct={'Disabled', 'Enabled'}  vector_style=Wide Row  use_help_units=off  help=''  units=''  use_header_enum=off  row_header_enum={}  col_header_enum={}  use_min_max=off  min_val=-inf  max_val=inf  use_precision=off  precision=''  gain=1  offset=0  exp=1  use_mototune_group=off  mototune_group=motohawk_vardec_path(gcb)
  motohawk_probe5 : MotoHawk_lib/Calibration & Probing Blocks/motohawk_probe  nam='EngineBlendfactor'  show_more=off  name_source=Use Parameter  read_level=1  view_as=Number  enum_struct={'Disabled', 'Enabled'}  vector_style=Wide Row  use_help_units=off  help=''  units=''  use_header_enum=off  row_header_enum={}  col_header_enum={}  use_min_max=off  min_val=-inf  max_val=inf  use_precision=off  precision=''  gain=1  offset=0  exp=1  use_mototune_group=off  mototune_group=motohawk_vardec_path(gcb)
  motohawk_probe6 : MotoHawk_lib/Calibration & Probing Blocks/motohawk_probe  nam='MotorBlendFactor'  show_more=off  name_source=Use Parameter  read_level=1  view_as=Number  enum_struct={'Disabled', 'Enabled'}  vector_style=Wide Row  use_help_units=off  help=''  units=''  use_header_enum=off  row_header_enum={}  col_header_enum={}  use_min_max=off  min_val=-inf  max_val=inf  use_precision=off  precision=''  gain=1  offset=0  exp=1  use_mototune_group=off  mototune_group=motohawk_vardec_path(gcb)
  motohawk_probe8 : MotoHawk_lib/Calibration & Probing Blocks/motohawk_probe  nam='Coil2'  show_more=off  name_source=Use Parameter  read_level=1  view_as=Number  enum_struct={'Disabled', 'Enabled'}  vector_style=Wide Row  use_help_units=off  help=''  units=''  use_header_enum=off  row_header_enum={}  col_header_enum={}  use_min_max=off  min_val=-inf  max_val=inf  use_precision=off  precision=''  gain=1  offset=0  exp=1  use_mototune_group=off  mototune_group=motohawk_vardec_path(gcb)
  motohawk_probe9 : MotoHawk_lib/Calibration & Probing Blocks/motohawk_probe  nam='MotortorqueReq'  show_more=off  name_source=Use Parameter  read_level=1  view_as=Number  enum_struct={'Disabled', 'Enabled'}  vector_style=Wide Row  use_help_units=off  help=''  units=''  use_header_enum=off  row_header_enum={}  col_header_enum={}  use_min_max=off  min_val=-inf  max_val=inf  use_precision=off  precision=''  gain=1  offset=0  exp=1  use_mototune_group=off  mototune_group=motohawk_vardec_path(gcb)
  motohawk_pwm : MotoHawk_lib/Analog I//O Blocks/motohawk_pwm  res_name=[]  text_resource=EST 1  target=ECU565-128  freq_mode=-1  min_freq=2  use_max_freq=off  max_freq=20000  use_enable=off  use_brake=off  output_current=on  output_fault_status=off  use_child=off  use_vardec=off  nam='PWMOutput'  read_level=1  write_level=1  group='System | I/O Pins | Outputs Config'
  wires:
  motohawk_calibration/1 -> Gain5/1
  Data Type Conversion3/1 -> motohawk_pwm/1
  Data Type Conversion11/1 -> motohawk_dout3/1, motohawk_probe15/1
  Data Type Conversion12/1 -> motohawk_probe11/1, motohawk_dout2/1
  Data Type Conversion13/1 -> motohawk_probe8/1, motohawk_dout1/1
  Data Type Conversion14/1 -> motohawk_probe3/1, motohawk_dout/1
  motohawk_pwm/1 -> Data Type Conversion16/1
  Data Type Conversion17/1 -> motohawk_dout4/1, motohawk_probe13/1
  Data Type Conversion18/1 -> motohawk_dout5/1, motohawk_probe14/1
  Data Type Conversion19/1 -> motohawk_probe12/1, motohawk_dout6/1
  Data Type Conversion16/1 -> Gain7/1
  Gain7/1 -> Data Type Conversion2/1, motohawk_probe16/1
  Gain1/1 -> Data Type Conversion3/1
  Data Type Conversion10/1 -> motohawk_pwm/2
  Gain5/1 -> Data Type Conversion10/1
  Data Type Conversion2/1 -> motohawk_dout7/1
  In14/1 -> Data Type Conversion11/1
  In2/1 -> motohawk_probe5/1
  In7/1 -> motohawk_probe10/1
  In8/1 -> Gain1/1, motohawk_probe9/1
  In1/1 -> Data Type Conversion19/1
  In4/1 -> motohawk_probe6/1
  In11/1 -> Data Type Conversion13/1
  In10/1 -> Data Type Conversion14/1
  In5/1 -> Data Type Conversion18/1
  In3/1 -> motohawk_probe1/1
  In6/1 -> Data Type Conversion17/1
  In12/1 -> Data Type Conversion12/1
  In13/1 -> motohawk_probe4/1

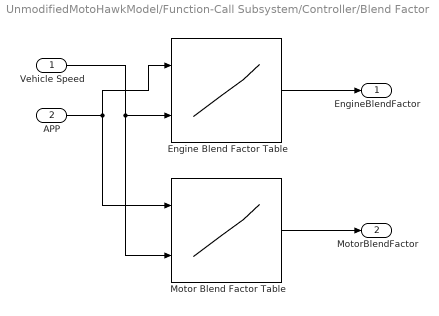
== system UnmodifiedMotoHawkModel/Function-Call Subsystem/Controller/Blend Factor ==
  Vehicle Speed : Inport
  APP : Inport  Port=2
  Engine Blend Factor Table : Lookup_n-D  BreakpointsForDimension1=v  BreakpointsForDimension2=x  Table=engineblendfactormap  InternalRulePriority=Speed  RndMeth=Simplest  InputSameDT=on
  Motor Blend Factor Table : Lookup_n-D  BreakpointsForDimension1=v  BreakpointsForDimension2=x  Table=motorblendfactormap  InternalRulePriority=Speed  RndMeth=Simplest  InputSameDT=on
  EngineBlendFactor : Outport
  MotorBlendFactor : Outport  Port=2
  wires:
  Engine Blend Factor Table/1 -> EngineBlendFactor/1
  Motor Blend Factor Table/1 -> MotorBlendFactor/1
  Vehicle Speed/1 -> Motor Blend Factor Table/2, Engine Blend Factor Table/2
  APP/1 -> Engine Blend Factor Table/1, Motor Blend Factor Table/1

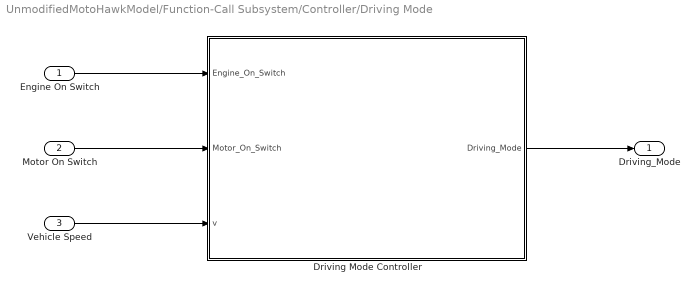
== system UnmodifiedMotoHawkModel/Function-Call Subsystem/Controller/Driving Mode ==
  Engine On Switch : Inport
  Motor On Switch : Inport  Port=2
  Vehicle Speed : Inport  Port=3
  Driving Mode Controller : Stateflow chart  TreatAsAtomicUnit=on
  Driving_Mode : Outport
  wires:
  Engine On Switch/1 -> Driving Mode Controller/1(Engine_On_Switch)
  Motor On Switch/1 -> Driving Mode Controller/2(Motor_On_Switch)
  Driving Mode Controller/1(Driving_Mode) -> Driving_Mode/1
  Vehicle Speed/1 -> Driving Mode Controller/3(v)

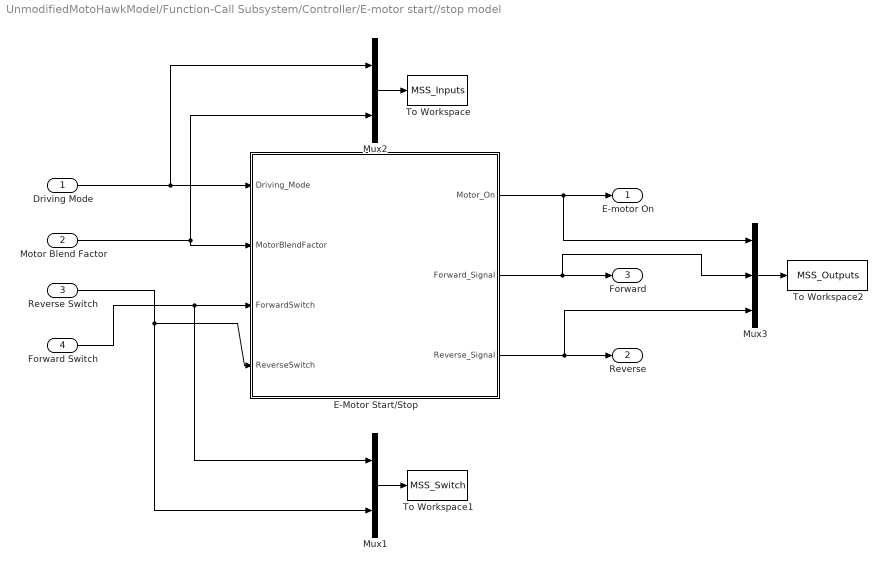
== system UnmodifiedMotoHawkModel/Function-Call Subsystem/Controller/E-motor start//stop model ==
  Driving Mode : Inport
  Motor Blend Factor : Inport  Port=2
  Reverse Switch : Inport  Port=3
  Forward Switch : Inport  Port=4
  E-Motor Start/Stop : Stateflow chart  TreatAsAtomicUnit=on
  Mux1 : Mux  Inputs=2
  Mux2 : Mux  Inputs=2
  Mux3 : Mux  Inputs=3
  To Workspace : ToWorkspace  VariableName=MSS_Inputs  SaveFormat=Structure With Time  SampleTime=-1
  To Workspace1 : ToWorkspace  VariableName=MSS_Switch  SaveFormat=Structure With Time  SampleTime=-1
  To Workspace2 : ToWorkspace  VariableName=MSS_Outputs  SaveFormat=Structure With Time  SampleTime=-1
  E-motor On : Outport
  Reverse : Outport  Port=2
  Forward : Outport  Port=3
  wires:
  Motor Blend Factor/1 -> E-Motor Start/Stop/2(MotorBlendFactor), Mux2/2
  Reverse Switch/1 -> Mux1/2, E-Motor Start/Stop/4(ReverseSwitch)
  Driving Mode/1 -> Mux2/1, E-Motor Start/Stop/1(Driving_Mode)
  Forward Switch/1 -> Mux1/1, E-Motor Start/Stop/3(ForwardSwitch)
  E-Motor Start/Stop/3(Reverse_Signal) -> Mux3/3, Reverse/1
  E-Motor Start/Stop/1(Motor_On) -> Mux3/1, E-motor On/1
  E-Motor Start/Stop/2(Forward_Signal) -> Mux3/2, Forward/1
  Mux2/1 -> To Workspace/1
  Mux1/1 -> To Workspace1/1
  Mux3/1 -> To Workspace2/1

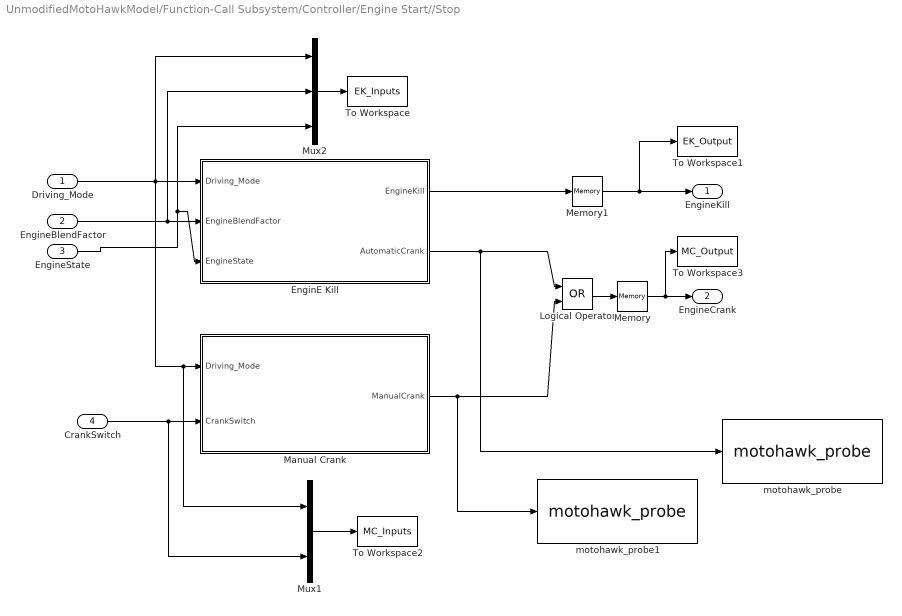
== system UnmodifiedMotoHawkModel/Function-Call Subsystem/Controller/Engine Start//Stop ==
  Driving_Mode : Inport
  EngineBlendFactor : Inport  Port=2
  EngineState : Inport  Port=3
  CrankSwitch : Inport  Port=4
  EnginE Kill : Stateflow chart  TreatAsAtomicUnit=on
  Logical Operator : Logic  Operator=OR  AllPortsSameDT=off  OutDataTypeStr=boolean
  Manual Crank : Stateflow chart  TreatAsAtomicUnit=on
  Memory : Memory  InheritSampleTime=on
  Memory1 : Memory  InheritSampleTime=on
  Mux1 : Mux  Inputs=2
  Mux2 : Mux  Inputs=3
  To Workspace : ToWorkspace  VariableName=EK_Inputs  SaveFormat=Structure With Time  SampleTime=-1
  To Workspace1 : ToWorkspace  VariableName=EK_Output  SaveFormat=Structure With Time  SampleTime=-1
  To Workspace2 : ToWorkspace  VariableName=MC_Inputs  SaveFormat=Structure With Time  SampleTime=-1
  To Workspace3 : ToWorkspace  VariableName=MC_Output  SaveFormat=Structure With Time  SampleTime=-1
  motohawk_probe : MotoHawk_lib/Calibration & Probing Blocks/motohawk_probe  nam='AutomaticCrank'  show_more=off  name_source=Use Parameter  read_level=1  view_as=Number  enum_struct={'Disabled', 'Enabled'}  vector_style=Wide Row  use_help_units=off  help=''  units=''  use_header_enum=off  row_header_enum={}  col_header_enum={}  use_min_max=off  min_val=-inf  max_val=inf  use_precision=off  precision=''  gain=1  offset=0  exp=1  use_mototune_group=off  mototune_group=motohawk_vardec_path(gcb)
  motohawk_probe1 : MotoHawk_lib/Calibration & Probing Blocks/motohawk_probe  nam='ManualCrank'  show_more=off  name_source=Use Parameter  read_level=1  view_as=Number  enum_struct={'Disabled', 'Enabled'}  vector_style=Wide Row  use_help_units=off  help=''  units=''  use_header_enum=off  row_header_enum={}  col_header_enum={}  use_min_max=off  min_val=-inf  max_val=inf  use_precision=off  precision=''  gain=1  offset=0  exp=1  use_mototune_group=off  mototune_group=motohawk_vardec_path(gcb)
  EngineKill : Outport
  EngineCrank : Outport  Port=2
  wires:
  EnginE Kill/2(AutomaticCrank) -> motohawk_probe/1, Logical Operator/1
  CrankSwitch/1 -> Mux1/2, Manual Crank/2(CrankSwitch)
  EngineBlendFactor/1 -> Mux2/2, EnginE Kill/2(EngineBlendFactor)
  EngineState/1 -> EnginE Kill/3(EngineState), Mux2/3
  EnginE Kill/1(EngineKill) -> Memory1/1
  Driving_Mode/1 -> Mux2/1, Mux1/1, Manual Crank/1(Driving_Mode), EnginE Kill/1(Driving_Mode)
  Manual Crank/1(ManualCrank) -> motohawk_probe1/1, Logical Operator/2
  Logical Operator/1 -> Memory/1
  Mux2/1 -> To Workspace/1
  Mux1/1 -> To Workspace2/1
  Memory/1 -> To Workspace3/1, EngineCrank/1
  Memory1/1 -> To Workspace1/1, EngineKill/1

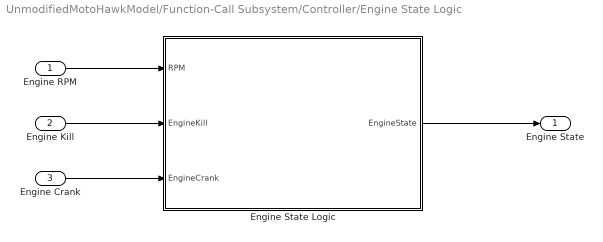
== system UnmodifiedMotoHawkModel/Function-Call Subsystem/Controller/Engine State Logic ==
  Engine RPM : Inport
  Engine Kill : Inport  Port=2
  Engine Crank : Inport  Port=3
  Engine State Logic : Stateflow chart  TreatAsAtomicUnit=on
  Engine State : Outport
  wires:
  Engine Kill/1 -> Engine State Logic/2(EngineKill)
  Engine RPM/1 -> Engine State Logic/1(RPM)
  Engine Crank/1 -> Engine State Logic/3(EngineCrank)
  Engine State Logic/1(EngineState) -> Engine State/1

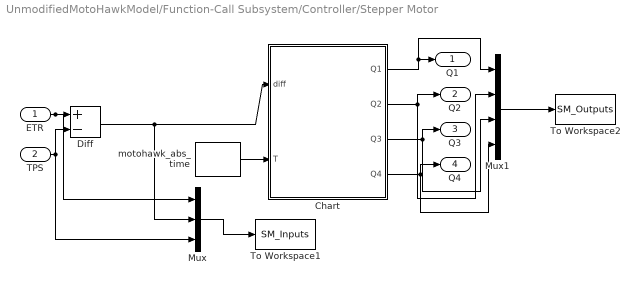
== system UnmodifiedMotoHawkModel/Function-Call Subsystem/Controller/Stepper Motor ==
  ETR : Inport
  TPS : Inport  Port=2
  Chart : Stateflow chart  TreatAsAtomicUnit=on
  Diff : Sum  Inputs=+-
  Mux : Mux  Inputs=3
  Mux1 : Mux
  To Workspace1 : ToWorkspace  VariableName=SM_Inputs  SaveFormat=Structure With Time  SampleTime=-1
  To Workspace2 : ToWorkspace  VariableName=SM_Outputs  SaveFormat=Structure With Time  SampleTime=-1
  motohawk_abs_time : MotoHawk_lib/Extra Development Blocks/motohawk_abs_time  mode=Seconds (double)  width=64 bit
  Q1 : Outport
  Q2 : Outport  Port=2
  Q3 : Outport  Port=3
  Q4 : Outport  Port=4
  wires:
  TPS/1 -> Mux/3, Diff/2
  Chart/2(Q2) -> Q2/1, Mux1/2
  Chart/3(Q3) -> Q3/1, Mux1/3
  Chart/4(Q4) -> Q4/1, Mux1/4
  Chart/1(Q1) -> Mux1/1, Q1/1
  ETR/1 -> Mux/1, Diff/1
  Diff/1 -> Mux/2, Chart/1(diff)
  Mux/1 -> To Workspace1/1
  Mux1/1 -> To Workspace2/1
  motohawk_abs_time/1 -> Chart/2(T)

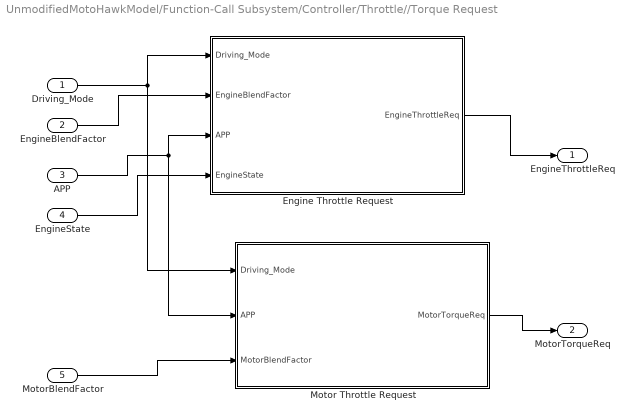
== system UnmodifiedMotoHawkModel/Function-Call Subsystem/Controller/Throttle//Torque Request ==
  Driving_Mode : Inport
  EngineBlendFactor : Inport  Port=2
  APP : Inport  Port=3
  EngineState : Inport  Port=4
  MotorBlendFactor : Inport  Port=5
  Engine Throttle Request : Stateflow chart  TreatAsAtomicUnit=on
  Motor Throttle Request : Stateflow chart  TreatAsAtomicUnit=on
  EngineThrottleReq : Outport
  MotorTorqueReq : Outport  Port=2
  wires:
  Driving_Mode/1 -> Motor Throttle Request/1(Driving_Mode), Engine Throttle Request/1(Driving_Mode)
  MotorBlendFactor/1 -> Motor Throttle Request/3(MotorBlendFactor)
  Engine Throttle Request/1(EngineThrottleReq) -> EngineThrottleReq/1
  Motor Throttle Request/1(MotorTorqueReq) -> MotorTorqueReq/1
  APP/1 -> Engine Throttle Request/3(APP), Motor Throttle Request/2(APP)
  EngineBlendFactor/1 -> Engine Throttle Request/2(EngineBlendFactor)
  EngineState/1 -> Engine Throttle Request/4(EngineState)
